simulink model "case1"  (R2024b)
settings: Solver=FixedStepAuto  StartTime=0  StopTime=1  FixedStep=1e-7  RelTol=1e-3
values from neighbouring files (symbols this model uses):
  SG_D_1_D = 0.01056    [IEEE9_case_parameters.m]    (also in case1_parameters.m; case2_parameters.m; case3_parameters.m; case4_parameters.m)
  SG_D_1_EnableSaturation = 0    [IEEE9_case_parameters.m]    (also in case1_parameters.m; case2_parameters.m; case3_parameters.m; case4_parameters.m)
  SG_D_1_f0 = 60    [IEEE9_case_parameters.m]    (also in case1_parameters.m; case2_parameters.m; case3_parameters.m; case4_parameters.m)
  SG_D_1_H = 7.5    [IEEE9_case_parameters.m]    (also in case1_parameters.m; case2_parameters.m; case3_parameters.m; case4_parameters.m)
  SG_D_1_K_A = 20    [IEEE9_case_parameters.m]    (also in case1_parameters.m; case2_parameters.m; case3_parameters.m; case4_parameters.m)
  SG_D_1_K_E = 1.000000e+1    (= 10)    [IEEE9_case_parameters.m]    (also in case1_parameters.m; case2_parameters.m; case3_parameters.m; case4_parameters.m)
  SG_D_1_K_F = 2.363    [IEEE9_case_parameters.m]    (also in case1_parameters.m; case2_parameters.m; case3_parameters.m; case4_parameters.m)
  SG_D_1_K_s = 0.5    [IEEE9_case_parameters.m]    (also in case1_parameters.m = 5; case2_parameters.m = 5; case3_parameters.m = 5; case4_parameters.m = 5)
  SG_D_1_R_a = 0.001088    [IEEE9_case_parameters.m]    (also in case1_parameters.m; case2_parameters.m; case3_parameters.m; case4_parameters.m)
  SG_D_1_S_A = 1    [IEEE9_case_parameters.m]    (also in case1_parameters.m; case2_parameters.m; case3_parameters.m; case4_parameters.m)
  SG_D_1_S_B = 0.103    [IEEE9_case_parameters.m]    (also in case1_parameters.m; case2_parameters.m; case3_parameters.m; case4_parameters.m)
  SG_D_1_S_N = 10.659857    [IEEE9_case_parameters.m]    (also in case1_parameters.m; case2_parameters.m; case3_parameters.m; case4_parameters.m)
  SG_D_1_SpeedPara = 200    [IEEE9_case_parameters.m]    (also in case1_parameters.m; case2_parameters.m; case3_parameters.m; case4_parameters.m)
  SG_D_1_T_0 = 0.720173    [IEEE9_case_parameters.m]    (also in case1_parameters.m = 0.755522; case2_parameters.m = 0.808931; case3_parameters.m = 0.869402; case4_parameters.m = 0.729316)
  SG_D_1_T_1 = 0.3    [IEEE9_case_parameters.m]    (also in case1_parameters.m; case2_parameters.m; case3_parameters.m; case4_parameters.m)
  SG_D_1_T_2 = 0.05    [IEEE9_case_parameters.m]    (also in case1_parameters.m; case2_parameters.m; case3_parameters.m; case4_parameters.m)
  SG_D_1_T_3 = 0.02    [IEEE9_case_parameters.m]    (also in case1_parameters.m; case2_parameters.m; case3_parameters.m; case4_parameters.m)
  SG_D_1_T_4 = 0.005    [IEEE9_case_parameters.m]    (also in case1_parameters.m; case2_parameters.m; case3_parameters.m; case4_parameters.m)
  SG_D_1_T_A = 0.02    [IEEE9_case_parameters.m]    (also in case1_parameters.m; case2_parameters.m; case3_parameters.m; case4_parameters.m)
  SG_D_1_T_dd = 8.000000e+0    (= 8)    [IEEE9_case_parameters.m]    (also in case1_parameters.m; case2_parameters.m; case3_parameters.m; case4_parameters.m)
  SG_D_1_T_ddd = 0.04    [IEEE9_case_parameters.m]    (also in case1_parameters.m; case2_parameters.m; case3_parameters.m; case4_parameters.m)
  SG_D_1_T_E = 0.314    [IEEE9_case_parameters.m]    (also in case1_parameters.m; case2_parameters.m; case3_parameters.m; case4_parameters.m)
  SG_D_1_T_F = 0.35    [IEEE9_case_parameters.m]    (also in case1_parameters.m; case2_parameters.m; case3_parameters.m; case4_parameters.m)
  SG_D_1_T_qd = 0.8    [IEEE9_case_parameters.m]    (also in case1_parameters.m; case2_parameters.m; case3_parameters.m; case4_parameters.m)
  SG_D_1_T_qdd = 0.02    [IEEE9_case_parameters.m]    (also in case1_parameters.m; case2_parameters.m; case3_parameters.m; case4_parameters.m)
  SG_D_1_T_speed = 0.1    [IEEE9_case_parameters.m]    (also in case1_parameters.m = 200; case2_parameters.m = 200; case3_parameters.m = 200; case4_parameters.m = 200)
  SG_D_1_T_w = 0.5    [IEEE9_case_parameters.m]    (also in case1_parameters.m; case2_parameters.m; case3_parameters.m; case4_parameters.m)
  SG_D_1_V_ref = 1.990276    [IEEE9_case_parameters.m]    (also in case1_parameters.m = 2.042296; case2_parameters.m = 2.051388; case3_parameters.m = 2.089584; case4_parameters.m = 2.01845)
  SG_D_1_w_ref = 376.991118    [IEEE9_case_parameters.m]    (also in case1_parameters.m; case2_parameters.m; case3_parameters.m; case4_parameters.m)
  SG_D_1_wb = 6.000000e+1    (= 60)    [IEEE9_case_parameters.m]    (also in case1_parameters.m; case2_parameters.m; case3_parameters.m; case4_parameters.m)
  SG_D_1_x_d = 1.9    [IEEE9_case_parameters.m]    (also in case1_parameters.m; case2_parameters.m; case3_parameters.m; case4_parameters.m)
  SG_D_1_x_dd = 0.302    [IEEE9_case_parameters.m]    (also in case1_parameters.m; case2_parameters.m; case3_parameters.m; case4_parameters.m)
  SG_D_1_x_ddd = 0.204    [IEEE9_case_parameters.m]    (also in case1_parameters.m; case2_parameters.m; case3_parameters.m; case4_parameters.m)
  SG_D_1_x_l = 0.05    [IEEE9_case_parameters.m]    (also in case1_parameters.m; case2_parameters.m; case3_parameters.m; case4_parameters.m)
  SG_D_1_x_q = 1.3    [IEEE9_case_parameters.m]    (also in case1_parameters.m; case2_parameters.m; case3_parameters.m; case4_parameters.m)
  SG_D_1_x_qd = 0.5    [IEEE9_case_parameters.m]    (also in case1_parameters.m; case2_parameters.m; case3_parameters.m; case4_parameters.m)
  SG_D_1_x_qdd = 0.3    [IEEE9_case_parameters.m]    (also in case1_parameters.m; case2_parameters.m; case3_parameters.m; case4_parameters.m)
  SG_D_2_D = 0.02    [IEEE9_case_parameters.m]    (also in case1_parameters.m; case2_parameters.m; case3_parameters.m; case4_parameters.m)
  SG_D_2_EnableSaturation = 0    [IEEE9_case_parameters.m]    (also in case1_parameters.m; case2_parameters.m; case3_parameters.m; case4_parameters.m)
  SG_D_2_f0 = 60    [IEEE9_case_parameters.m]    (also in case1_parameters.m; case2_parameters.m; case3_parameters.m; case4_parameters.m)
  SG_D_2_H = 8.000000e+0    (= 8)    [IEEE9_case_parameters.m]    (also in case1_parameters.m; case2_parameters.m; case3_parameters.m; case4_parameters.m)
  SG_D_2_K_A = 20    [IEEE9_case_parameters.m]    (also in case1_parameters.m; case2_parameters.m; case3_parameters.m; case4_parameters.m)
  SG_D_2_K_E = 1.000000e+1    (= 10)    [IEEE9_case_parameters.m]    (also in case1_parameters.m; case2_parameters.m; case3_parameters.m; case4_parameters.m)
  SG_D_2_K_F = 2.363    [IEEE9_case_parameters.m]    (also in case1_parameters.m; case2_parameters.m; case3_parameters.m; case4_parameters.m)
  SG_D_2_K_s = 0.5    [IEEE9_case_parameters.m]    (also in case1_parameters.m = 4; case2_parameters.m = 4; case3_parameters.m = 4; case4_parameters.m = 4)
  SG_D_2_R_a = 0.001088    [IEEE9_case_parameters.m]    (also in case1_parameters.m; case2_parameters.m; case3_parameters.m; case4_parameters.m)
  SG_D_2_S_A = 1    [IEEE9_case_parameters.m]    (also in case1_parameters.m; case2_parameters.m; case3_parameters.m; case4_parameters.m)
  SG_D_2_S_B = 0.103    [IEEE9_case_parameters.m]    (also in case1_parameters.m; case2_parameters.m; case3_parameters.m; case4_parameters.m)
  SG_D_2_S_N = 10.659857    [IEEE9_case_parameters.m]    (also in case1_parameters.m; case2_parameters.m; case3_parameters.m; case4_parameters.m)
  SG_D_2_SpeedPara = 200    [IEEE9_case_parameters.m]    (also in case1_parameters.m; case2_parameters.m; case3_parameters.m; case4_parameters.m)
  SG_D_2_T_0 = 1.632913    [IEEE9_case_parameters.m]    (also in case1_parameters.m = 1.632925; case2_parameters.m = 1.632915; case3_parameters.m = 1.632914; case4_parameters.m = 1.632927)
  SG_D_2_T_1 = 0.2    [IEEE9_case_parameters.m]    (also in case1_parameters.m; case2_parameters.m; case3_parameters.m; case4_parameters.m)
  SG_D_2_T_2 = 0.05    [IEEE9_case_parameters.m]    (also in case1_parameters.m; case2_parameters.m; case3_parameters.m; case4_parameters.m)
  SG_D_2_T_3 = 0.02    [IEEE9_case_parameters.m]    (also in case1_parameters.m; case2_parameters.m; case3_parameters.m; case4_parameters.m)
  SG_D_2_T_4 = 0.005    [IEEE9_case_parameters.m]    (also in case1_parameters.m; case2_parameters.m; case3_parameters.m; case4_parameters.m)
  SG_D_2_T_A = 0.02    [IEEE9_case_parameters.m]    (also in case1_parameters.m; case2_parameters.m; case3_parameters.m; case4_parameters.m)
  SG_D_2_T_dd = 7.9    [IEEE9_case_parameters.m]    (also in case1_parameters.m; case2_parameters.m; case3_parameters.m; case4_parameters.m)
  SG_D_2_T_ddd = 0.04    [IEEE9_case_parameters.m]    (also in case1_parameters.m; case2_parameters.m; case3_parameters.m; case4_parameters.m)
  SG_D_2_T_E = 0.314    [IEEE9_case_parameters.m]    (also in case1_parameters.m; case2_parameters.m; case3_parameters.m; case4_parameters.m)
  SG_D_2_T_F = 0.35    [IEEE9_case_parameters.m]    (also in case1_parameters.m; case2_parameters.m; case3_parameters.m; case4_parameters.m)
  SG_D_2_T_qd = 0.8    [IEEE9_case_parameters.m]    (also in case1_parameters.m; case2_parameters.m; case3_parameters.m; case4_parameters.m)
  SG_D_2_T_qdd = 0.015    [IEEE9_case_parameters.m]    (also in case1_parameters.m; case2_parameters.m; case3_parameters.m; case4_parameters.m)
  SG_D_2_T_speed = 0.1    [IEEE9_case_parameters.m]    (also in case1_parameters.m = 150; case2_parameters.m = 150; case3_parameters.m = 150; case4_parameters.m = 150)
  SG_D_2_T_w = 0.35    [IEEE9_case_parameters.m]    (also in case1_parameters.m; case2_parameters.m; case3_parameters.m; case4_parameters.m)
  SG_D_2_V_ref = 2.58547    [IEEE9_case_parameters.m]    (also in case1_parameters.m = 2.597896; case2_parameters.m = 2.587136; case3_parameters.m = 2.586042; case4_parameters.m = 2.599679)
  SG_D_2_w_ref = 376.991118    [IEEE9_case_parameters.m]    (also in case1_parameters.m; case2_parameters.m; case3_parameters.m; case4_parameters.m)
  SG_D_2_wb = 6.000000e+1    (= 60)    [IEEE9_case_parameters.m]    (also in case1_parameters.m; case2_parameters.m; case3_parameters.m; case4_parameters.m)
  SG_D_2_x_d = 1.8    [IEEE9_case_parameters.m]    (also in case1_parameters.m; case2_parameters.m; case3_parameters.m; case4_parameters.m)
  SG_D_2_x_dd = 0.302    [IEEE9_case_parameters.m]    (also in case1_parameters.m; case2_parameters.m; case3_parameters.m; case4_parameters.m)
  SG_D_2_x_ddd = 0.204    [IEEE9_case_parameters.m]    (also in case1_parameters.m; case2_parameters.m; case3_parameters.m; case4_parameters.m)
  SG_D_2_x_l = 0.05    [IEEE9_case_parameters.m]    (also in case1_parameters.m; case2_parameters.m; case3_parameters.m; case4_parameters.m)
  SG_D_2_x_q = 1.25    [IEEE9_case_parameters.m]    (also in case1_parameters.m; case2_parameters.m; case3_parameters.m; case4_parameters.m)
  SG_D_2_x_qd = 0.5    [IEEE9_case_parameters.m]    (also in case1_parameters.m; case2_parameters.m; case3_parameters.m; case4_parameters.m)
  SG_D_2_x_qdd = 0.3    [IEEE9_case_parameters.m]    (also in case1_parameters.m; case2_parameters.m; case3_parameters.m; case4_parameters.m)
  SG_D_3_D = 0.02    [IEEE9_case_parameters.m]    (also in case1_parameters.m; case2_parameters.m; case3_parameters.m; case4_parameters.m)
  SG_D_3_EnableSaturation = 0    [IEEE9_case_parameters.m]    (also in case1_parameters.m; case2_parameters.m; case3_parameters.m; case4_parameters.m)
  SG_D_3_f0 = 60    [IEEE9_case_parameters.m]    (also in case1_parameters.m; case2_parameters.m; case3_parameters.m; case4_parameters.m)
  SG_D_3_H = 7.7    [IEEE9_case_parameters.m]    (also in case1_parameters.m; case2_parameters.m; case3_parameters.m; case4_parameters.m)
  SG_D_3_K_A = 20    [IEEE9_case_parameters.m]    (also in case1_parameters.m; case2_parameters.m; case3_parameters.m; case4_parameters.m)
  SG_D_3_K_E = 1.000000e+1    (= 10)    [IEEE9_case_parameters.m]    (also in case1_parameters.m; case2_parameters.m; case3_parameters.m; case4_parameters.m)
  SG_D_3_K_F = 2.363    [IEEE9_case_parameters.m]    (also in case1_parameters.m; case2_parameters.m; case3_parameters.m; case4_parameters.m)
  SG_D_3_K_s = 0.2    [IEEE9_case_parameters.m]    (also in case1_parameters.m = 2; case2_parameters.m = 2; case3_parameters.m = 2; case4_parameters.m = 2)
  SG_D_3_R_a = 0.001088    [IEEE9_case_parameters.m]    (also in case1_parameters.m; case2_parameters.m; case3_parameters.m; case4_parameters.m)
  SG_D_3_S_A = 1    [IEEE9_case_parameters.m]    (also in case1_parameters.m; case2_parameters.m; case3_parameters.m; case4_parameters.m)
  SG_D_3_S_B = 0.103    [IEEE9_case_parameters.m]    (also in case1_parameters.m; case2_parameters.m; case3_parameters.m; case4_parameters.m)
  SG_D_3_S_N = 10.659857    [IEEE9_case_parameters.m]    (also in case1_parameters.m; case2_parameters.m; case3_parameters.m; case4_parameters.m)
  SG_D_3_SpeedPara = 200    [IEEE9_case_parameters.m]    (also in case1_parameters.m; case2_parameters.m; case3_parameters.m; case4_parameters.m)
  SG_D_3_T_0 = 0.850788    [IEEE9_case_parameters.m]    (also in case1_parameters.m = 0.850786; case2_parameters.m = 0.850787; case3_parameters.m; case4_parameters.m = 0.850786)
  SG_D_3_T_1 = 0.2    [IEEE9_case_parameters.m]    (also in case1_parameters.m; case2_parameters.m; case3_parameters.m; case4_parameters.m)
  SG_D_3_T_2 = 0.05    [IEEE9_case_parameters.m]    (also in case1_parameters.m; case2_parameters.m; case3_parameters.m; case4_parameters.m)
  SG_D_3_T_3 = 0.02    [IEEE9_case_parameters.m]    (also in case1_parameters.m; case2_parameters.m; case3_parameters.m; case4_parameters.m)
  SG_D_3_T_4 = 0.005    [IEEE9_case_parameters.m]    (also in case1_parameters.m; case2_parameters.m; case3_parameters.m; case4_parameters.m)
  SG_D_3_T_A = 0.02    [IEEE9_case_parameters.m]    (also in case1_parameters.m; case2_parameters.m; case3_parameters.m; case4_parameters.m)
  SG_D_3_T_dd = 8.1    [IEEE9_case_parameters.m]    (also in case1_parameters.m; case2_parameters.m; case3_parameters.m; case4_parameters.m)
  SG_D_3_T_ddd = 0.04    [IEEE9_case_parameters.m]    (also in case1_parameters.m; case2_parameters.m; case3_parameters.m; case4_parameters.m)
  SG_D_3_T_E = 0.314    [IEEE9_case_parameters.m]    (also in case1_parameters.m; case2_parameters.m; case3_parameters.m; case4_parameters.m)
  SG_D_3_T_F = 0.35    [IEEE9_case_parameters.m]    (also in case1_parameters.m; case2_parameters.m; case3_parameters.m; case4_parameters.m)
  SG_D_3_T_qd = 0.8    [IEEE9_case_parameters.m]    (also in case1_parameters.m; case2_parameters.m; case3_parameters.m; case4_parameters.m)
  SG_D_3_T_qdd = 0.015    [IEEE9_case_parameters.m]    (also in case1_parameters.m; case2_parameters.m; case3_parameters.m; case4_parameters.m)
  SG_D_3_T_speed = 0.1    [IEEE9_case_parameters.m]    (also in case1_parameters.m = 180; case2_parameters.m = 180; case3_parameters.m = 180; case4_parameters.m = 180)
  SG_D_3_T_w = 0.4    [IEEE9_case_parameters.m]    (also in case1_parameters.m; case2_parameters.m; case3_parameters.m; case4_parameters.m)
  SG_D_3_V_ref = 1.892727    [IEEE9_case_parameters.m]    (also in case1_parameters.m = 1.906439; case2_parameters.m = 1.895535; case3_parameters.m = 1.892105; case4_parameters.m = 1.906598)
  SG_D_3_w_ref = 376.991118    [IEEE9_case_parameters.m]    (also in case1_parameters.m; case2_parameters.m; case3_parameters.m; case4_parameters.m)
  SG_D_3_wb = 6.000000e+1    (= 60)    [IEEE9_case_parameters.m]    (also in case1_parameters.m; case2_parameters.m; case3_parameters.m; case4_parameters.m)
  SG_D_3_x_d = 1.85    [IEEE9_case_parameters.m]    (also in case1_parameters.m; case2_parameters.m; case3_parameters.m; case4_parameters.m)
  SG_D_3_x_dd = 0.302    [IEEE9_case_parameters.m]    (also in case1_parameters.m; case2_parameters.m; case3_parameters.m; case4_parameters.m)
  SG_D_3_x_ddd = 0.204    [IEEE9_case_parameters.m]    (also in case1_parameters.m; case2_parameters.m; case3_parameters.m; case4_parameters.m)
  SG_D_3_x_l = 0.05    [IEEE9_case_parameters.m]    (also in case1_parameters.m; case2_parameters.m; case3_parameters.m; case4_parameters.m)
  SG_D_3_x_q = 1.2    [IEEE9_case_parameters.m]    (also in case1_parameters.m; case2_parameters.m; case3_parameters.m; case4_parameters.m)
  SG_D_3_x_qd = 0.5    [IEEE9_case_parameters.m]    (also in case1_parameters.m; case2_parameters.m; case3_parameters.m; case4_parameters.m)
  SG_D_3_x_qdd = 0.3    [IEEE9_case_parameters.m]    (also in case1_parameters.m; case2_parameters.m; case3_parameters.m; case4_parameters.m)
(part 2 of 12)

== system case1/SG_D_2 ==
  v_d_SG_D_2 : Inport
  v_q_SG_D_2 : Inport  Port=2
  E_fd_SG_D_2 : Integrator  InitialCondition=3.195791296561274
  Px_1_SG_D_2 : Integrator  InitialCondition=0.0
  Px_2_SG_D_2 : Integrator  InitialCondition=0.0
  Px_3_SG_D_2 : Integrator  InitialCondition=7.086697555280228e-24
  R_f_SG_D_2 : Integrator  InitialCondition=21.576156667926544
  T_e_SG_D_2_block : Subsystem
  T_m_SG_D_2 : Integrator  InitialCondition=1.6329252190417882
  V_f_SG_D_2 : Integrator  InitialCondition=31.95791296561274
  d_E_fd_SG_D_2_block : Subsystem
  d_Px_1_SG_D_2_block : Subsystem
  d_Px_2_SG_D_2_block : Subsystem
  d_Px_3_SG_D_2_block : Subsystem
  d_R_f_SG_D_2_block : Subsystem
  d_T_m_SG_D_2_block : Subsystem
  d_V_f_SG_D_2_block : Subsystem
  d_psi_1d_SG_D_2_block : Subsystem
  d_psi_d_SG_D_2_block : Subsystem
  d_psi_fd_SG_D_2_block : Subsystem
  d_psi_gq_SG_D_2_block : Subsystem
  d_psi_kq_SG_D_2_block : Subsystem
  d_psi_q_SG_D_2_block : Subsystem
  d_theta_SG_D_2_block : Subsystem
  d_w_SG_D_2_block : Subsystem
  i_d_SG_D_2_block : Subsystem
  i_q_SG_D_2_block : Subsystem
  psi_1d_SG_D_2 : Integrator  InitialCondition=0.5903095464731192
  psi_d_SG_D_2 : Integrator  InitialCondition=0.5158672107563145
  psi_fd_SG_D_2 : Integrator  InitialCondition=0.9654989184858135
  psi_gq_SG_D_2 : Integrator  InitialCondition=0.5152428462796697
  psi_kq_SG_D_2 : Integrator  InitialCondition=-0.8243885540474714
  psi_q_SG_D_2 : Integrator  InitialCondition=-0.8587380771327827
  theta_SG_D_2 : Integrator  InitialCondition=1.1983532874479317
  theta_SG_D_2_out_block : Subsystem
  w_SG_D_2 : Integrator  InitialCondition=376.99111843077515
  w_SG_D_2_out_block : Subsystem
  i_d_SG_D_2 : Outport
  i_q_SG_D_2 : Outport  Port=2
  T_e_SG_D_2 : Outport  Port=3
  w_SG_D_2_out : Outport  Port=4
  theta_SG_D_2_out : Outport  Port=5
  wires:
  d_T_m_SG_D_2_block/1(Blockout_d_T_m_SG_D_2_43af5) -> T_m_SG_D_2/1
  T_e_SG_D_2_block/1(Blockout_T_e_SG_D_2_b65d9) -> T_e_SG_D_2/1
  d_Px_2_SG_D_2_block/1(Blockout_d_Px_2_SG_D_2_74daf) -> Px_2_SG_D_2/1
  w_SG_D_2/1 -> d_psi_d_SG_D_2_block/9(State_w_SG_D_2_46e5d), d_w_SG_D_2_block/1(State_w_SG_D_2_d69c3), d_V_f_SG_D_2_block/13(State_w_SG_D_2_2be4f), d_psi_q_SG_D_2_block/9(State_w_SG_D_2_df282), d_theta_SG_D_2_block/1(State_w_SG_D_2_5c0a1), d_Px_1_SG_D_2_block/2(State_w_SG_D_2_a2171), d_T_m_SG_D_2_block/1(State_w_SG_D_2_723fe), d_Px_3_SG_D_2_block/6(State_w_SG_D_2_a0c55), d_Px_2_SG_D_2_block/4(State_w_SG_D_2_d1507), d_V_f_SG_D_2_block/8(State_w_SG_D_2_bb1ed), w_SG_D_2_out_block/1(State_w_SG_D_2_39d84)
  d_Px_1_SG_D_2_block/1(Blockout_d_Px_1_SG_D_2_8641a) -> Px_1_SG_D_2/1
  d_theta_SG_D_2_block/1(Blockout_d_theta_SG_D_2_6c47c) -> theta_SG_D_2/1
  d_Px_3_SG_D_2_block/1(Blockout_d_Px_3_SG_D_2_3521b) -> Px_3_SG_D_2/1
  psi_q_SG_D_2/1 -> d_psi_d_SG_D_2_block/8(State_psi_q_SG_D_2_06491), d_psi_gq_SG_D_2_block/6(State_psi_q_SG_D_2_986ec), d_psi_gq_SG_D_2_block/9(State_psi_q_SG_D_2_b4e81), d_psi_kq_SG_D_2_block/5(State_psi_q_SG_D_2_af7b5), d_w_SG_D_2_block/6(State_psi_q_SG_D_2_041d5), d_V_f_SG_D_2_block/11(State_psi_q_SG_D_2_14f0d), d_psi_q_SG_D_2_block/3(State_psi_q_SG_D_2_34d65), i_d_SG_D_2_block/3(State_psi_q_SG_D_2_a8ffe), i_q_SG_D_2_block/3(State_psi_q_SG_D_2_008e1), T_e_SG_D_2_block/4(State_psi_q_SG_D_2_25b32), T_e_SG_D_2_block/5(State_psi_q_SG_D_2_fddea), d_V_f_SG_D_2_block/7(State_psi_q_SG_D_2_09452), d_w_SG_D_2_block/7(State_psi_q_SG_D_2_a083f)
  w_SG_D_2_out_block/1(Blockout_w_SG_D_2_out_2e2ba) -> w_SG_D_2_out/1
  psi_gq_SG_D_2/1 -> d_psi_q_SG_D_2_block/1(State_psi_gq_SG_D_2_52ba9), d_psi_gq_SG_D_2_block/2(State_psi_gq_SG_D_2_2d72f), d_psi_gq_SG_D_2_block/4(State_psi_gq_SG_D_2_96f10), d_V_f_SG_D_2_block/9(State_psi_gq_SG_D_2_56303), d_psi_gq_SG_D_2_block/1(State_psi_gq_SG_D_2_d4904), i_d_SG_D_2_block/1(State_psi_gq_SG_D_2_0a4ff), d_psi_kq_SG_D_2_block/3(State_psi_gq_SG_D_2_c1bff), d_psi_kq_SG_D_2_block/1(State_psi_gq_SG_D_2_b21d1), i_q_SG_D_2_block/1(State_psi_gq_SG_D_2_4b38b), d_w_SG_D_2_block/4(State_psi_gq_SG_D_2_37098), T_e_SG_D_2_block/2(State_psi_gq_SG_D_2_50ede), d_psi_gq_SG_D_2_block/7(State_psi_gq_SG_D_2_84d01)
  psi_fd_SG_D_2/1 -> d_psi_fd_SG_D_2_block/2(State_psi_fd_SG_D_2_87c43), d_psi_fd_SG_D_2_block/4(State_psi_fd_SG_D_2_c572b), d_psi_fd_SG_D_2_block/7(State_psi_fd_SG_D_2_150ec), d_psi_fd_SG_D_2_block/10(State_psi_fd_SG_D_2_9d902), d_psi_d_SG_D_2_block/3(State_psi_fd_SG_D_2_4d493), d_psi_1d_SG_D_2_block/5(State_psi_fd_SG_D_2_2bfe4), d_w_SG_D_2_block/10(State_psi_fd_SG_D_2_0ad40), d_psi_1d_SG_D_2_block/2(State_psi_fd_SG_D_2_d5601), i_d_SG_D_2_block/7(State_psi_fd_SG_D_2_62171), i_q_SG_D_2_block/7(State_psi_fd_SG_D_2_0701d), T_e_SG_D_2_block/8(State_psi_fd_SG_D_2_27f6e), d_V_f_SG_D_2_block/6(State_psi_fd_SG_D_2_7e9d1)
  Px_1_SG_D_2/1 -> d_Px_2_SG_D_2_block/2(State_Px_1_SG_D_2_4a486), d_Px_3_SG_D_2_block/4(State_Px_1_SG_D_2_19b2b), d_Px_3_SG_D_2_block/5(State_Px_1_SG_D_2_dcab9), d_Px_2_SG_D_2_block/3(State_Px_1_SG_D_2_0c9fb), d_Px_1_SG_D_2_block/1(State_Px_1_SG_D_2_dab25)
  psi_1d_SG_D_2/1 -> d_psi_fd_SG_D_2_block/3(State_psi_1d_SG_D_2_cf418), d_psi_fd_SG_D_2_block/5(State_psi_1d_SG_D_2_6822c), d_psi_fd_SG_D_2_block/8(State_psi_1d_SG_D_2_241cc), d_psi_d_SG_D_2_block/1(State_psi_1d_SG_D_2_48ea4), d_w_SG_D_2_block/8(State_psi_1d_SG_D_2_7d072), d_psi_1d_SG_D_2_block/3(State_psi_1d_SG_D_2_3af5a), d_psi_1d_SG_D_2_block/1(State_psi_1d_SG_D_2_96ec3), d_V_f_SG_D_2_block/4(State_psi_1d_SG_D_2_f4f15), i_d_SG_D_2_block/5(State_psi_1d_SG_D_2_a6845), i_q_SG_D_2_block/5(State_psi_1d_SG_D_2_4cf3f), T_e_SG_D_2_block/6(State_psi_1d_SG_D_2_6821c)
  i_d_SG_D_2_block/1(Blockout_i_d_SG_D_2_76c8b) -> i_d_SG_D_2/1
  psi_d_SG_D_2/1 -> d_psi_d_SG_D_2_block/2(State_psi_d_SG_D_2_8d25d), d_psi_1d_SG_D_2_block/4(State_psi_d_SG_D_2_4d81a), i_d_SG_D_2_block/6(State_psi_d_SG_D_2_bb259), d_psi_q_SG_D_2_block/8(State_psi_d_SG_D_2_1d0f8), d_V_f_SG_D_2_block/12(State_psi_d_SG_D_2_84408), d_psi_fd_SG_D_2_block/9(State_psi_d_SG_D_2_887e8), d_w_SG_D_2_block/9(State_psi_d_SG_D_2_8384e), d_w_SG_D_2_block/3(State_psi_d_SG_D_2_3a37a), i_q_SG_D_2_block/6(State_psi_d_SG_D_2_91eea), d_V_f_SG_D_2_block/5(State_psi_d_SG_D_2_39d83), d_psi_fd_SG_D_2_block/6(State_psi_d_SG_D_2_85721), T_e_SG_D_2_block/1(State_psi_d_SG_D_2_d17d7), T_e_SG_D_2_block/7(State_psi_d_SG_D_2_3bce2)
  psi_kq_SG_D_2/1 -> d_psi_q_SG_D_2_block/2(State_psi_kq_SG_D_2_a91e4), d_psi_gq_SG_D_2_block/3(State_psi_kq_SG_D_2_8efed), d_psi_gq_SG_D_2_block/5(State_psi_kq_SG_D_2_f03b3), d_psi_kq_SG_D_2_block/2(State_psi_kq_SG_D_2_91d69), d_psi_gq_SG_D_2_block/8(State_psi_kq_SG_D_2_c2c6b), d_psi_kq_SG_D_2_block/4(State_psi_kq_SG_D_2_611bb), i_d_SG_D_2_block/2(State_psi_kq_SG_D_2_7acfc), i_q_SG_D_2_block/2(State_psi_kq_SG_D_2_d6d60), d_V_f_SG_D_2_block/10(State_psi_kq_SG_D_2_82247), d_w_SG_D_2_block/5(State_psi_kq_SG_D_2_af83b), T_e_SG_D_2_block/3(State_psi_kq_SG_D_2_ad282)
  v_d_SG_D_2/1 -> d_psi_d_SG_D_2_block/4(Input_v_d_SG_D_2_e74d4), d_psi_q_SG_D_2_block/4(Input_v_d_SG_D_2_5ea16)
  T_m_SG_D_2/1 -> d_T_m_SG_D_2_block/2(State_T_m_SG_D_2_d95aa), d_w_SG_D_2_block/2(State_T_m_SG_D_2_7a8a9)
  d_V_f_SG_D_2_block/1(Blockout_d_V_f_SG_D_2_347d2) -> V_f_SG_D_2/1
  v_q_SG_D_2/1 -> d_psi_d_SG_D_2_block/6(Input_v_q_SG_D_2_ef7b1), d_psi_q_SG_D_2_block/6(Input_v_q_SG_D_2_1b817)
  Px_2_SG_D_2/1 -> d_Px_2_SG_D_2_block/1(State_Px_2_SG_D_2_5b382), d_Px_3_SG_D_2_block/3(State_Px_2_SG_D_2_7bb9c), d_Px_3_SG_D_2_block/2(State_Px_2_SG_D_2_29f59)
  theta_SG_D_2/1 -> d_psi_q_SG_D_2_block/5(State_theta_SG_D_2_2fc52), i_d_SG_D_2_block/8(State_theta_SG_D_2_f5053), i_q_SG_D_2_block/8(State_theta_SG_D_2_18733), i_q_SG_D_2_block/4(State_theta_SG_D_2_18eff), theta_SG_D_2_out_block/1(State_theta_SG_D_2_2515d), i_d_SG_D_2_block/4(State_theta_SG_D_2_c8d9f), d_psi_d_SG_D_2_block/7(State_theta_SG_D_2_069cc), d_psi_q_SG_D_2_block/7(State_theta_SG_D_2_f1308), d_psi_d_SG_D_2_block/5(State_theta_SG_D_2_cb884)
  d_psi_1d_SG_D_2_block/1(Blockout_d_psi_1d_SG_D_2_57022) -> psi_1d_SG_D_2/1
  d_R_f_SG_D_2_block/1(Blockout_d_R_f_SG_D_2_3f1f3) -> R_f_SG_D_2/1
  R_f_SG_D_2/1 -> d_V_f_SG_D_2_block/2(State_R_f_SG_D_2_e5370), d_R_f_SG_D_2_block/2(State_R_f_SG_D_2_6bf16)
  theta_SG_D_2_out_block/1(Blockout_theta_SG_D_2_out_503d1) -> theta_SG_D_2_out/1
  d_psi_gq_SG_D_2_block/1(Blockout_d_psi_gq_SG_D_2_f38dc) -> psi_gq_SG_D_2/1
  d_psi_d_SG_D_2_block/1(Blockout_d_psi_d_SG_D_2_591f5) -> psi_d_SG_D_2/1
  d_w_SG_D_2_block/1(Blockout_d_w_SG_D_2_dff9f) -> w_SG_D_2/1
  d_psi_q_SG_D_2_block/1(Blockout_d_psi_q_SG_D_2_5eec6) -> psi_q_SG_D_2/1
  d_psi_kq_SG_D_2_block/1(Blockout_d_psi_kq_SG_D_2_4ff78) -> psi_kq_SG_D_2/1
  i_q_SG_D_2_block/1(Blockout_i_q_SG_D_2_02eb4) -> i_q_SG_D_2/1
  V_f_SG_D_2/1 -> d_V_f_SG_D_2_block/14(State_V_f_SG_D_2_eb789), d_E_fd_SG_D_2_block/2(State_V_f_SG_D_2_853e9)
  Px_3_SG_D_2/1 -> d_V_f_SG_D_2_block/3(State_Px_3_SG_D_2_3a9e9), d_Px_3_SG_D_2_block/1(State_Px_3_SG_D_2_47d77)
  d_E_fd_SG_D_2_block/1(Blockout_d_E_fd_SG_D_2_6e556) -> E_fd_SG_D_2/1
  E_fd_SG_D_2/1 -> d_V_f_SG_D_2_block/1(State_E_fd_SG_D_2_4dd56), d_R_f_SG_D_2_block/1(State_E_fd_SG_D_2_b3245), d_psi_fd_SG_D_2_block/1(State_E_fd_SG_D_2_9c9d0), d_E_fd_SG_D_2_block/1(State_E_fd_SG_D_2_f3b44)
  d_psi_fd_SG_D_2_block/1(Blockout_d_psi_fd_SG_D_2_b0c7a) -> psi_fd_SG_D_2/1

== system case1/SG_D_3 ==
  v_d_SG_D_3 : Inport
  v_q_SG_D_3 : Inport  Port=2
  E_fd_SG_D_3 : Integrator  InitialCondition=1.8128770595240795
  Px_1_SG_D_3 : Integrator  InitialCondition=0.0
  Px_2_SG_D_3 : Integrator  InitialCondition=0.0
  Px_3_SG_D_3 : Integrator  InitialCondition=5.5764488625501145e-24
  R_f_SG_D_3 : Integrator  InitialCondition=12.239509976158287
  T_e_SG_D_3_block : Subsystem
  T_m_SG_D_3 : Integrator  InitialCondition=0.8507861887621803
  V_f_SG_D_3 : Integrator  InitialCondition=18.1287705952408
  d_E_fd_SG_D_3_block : Subsystem
  d_Px_1_SG_D_3_block : Subsystem
  d_Px_2_SG_D_3_block : Subsystem
  d_Px_3_SG_D_3_block : Subsystem
  d_R_f_SG_D_3_block : Subsystem
  d_T_m_SG_D_3_block : Subsystem
  d_V_f_SG_D_3_block : Subsystem
  d_psi_1d_SG_D_3_block : Subsystem
  d_psi_d_SG_D_3_block : Subsystem
  d_psi_fd_SG_D_3_block : Subsystem
  d_psi_gq_SG_D_3_block : Subsystem
  d_psi_kq_SG_D_3_block : Subsystem
  d_psi_q_SG_D_3_block : Subsystem
  d_theta_SG_D_3_block : Subsystem
  d_w_SG_D_3_block : Subsystem
  i_d_SG_D_3_block : Subsystem
  i_q_SG_D_3_block : Subsystem
  psi_1d_SG_D_3 : Integrator  InitialCondition=0.7269094989362452
  psi_d_SG_D_3 : Integrator  InitialCondition=0.6967437333643608
  psi_fd_SG_D_3 : Integrator  InitialCondition=0.8789449574185421
  psi_gq_SG_D_3 : Integrator  InitialCondition=0.419188473974919
  psi_kq_SG_D_3 : Integrator  InitialCondition=-0.6886667786730812
  psi_q_SG_D_3 : Integrator  InitialCondition=-0.7186088125284327
  theta_SG_D_3 : Integrator  InitialCondition=0.88169001906526
  theta_SG_D_3_out_block : Subsystem
  w_SG_D_3 : Integrator  InitialCondition=376.99111843077515
  w_SG_D_3_out_block : Subsystem
  i_d_SG_D_3 : Outport
  i_q_SG_D_3 : Outport  Port=2
  T_e_SG_D_3 : Outport  Port=3
  w_SG_D_3_out : Outport  Port=4
  theta_SG_D_3_out : Outport  Port=5
  wires:
  d_Px_1_SG_D_3_block/1(Blockout_d_Px_1_SG_D_3_617e0) -> Px_1_SG_D_3/1
  w_SG_D_3/1 -> d_V_f_SG_D_3_block/13(State_w_SG_D_3_e4083), d_w_SG_D_3_block/1(State_w_SG_D_3_f2997), d_V_f_SG_D_3_block/8(State_w_SG_D_3_c73a4), d_psi_d_SG_D_3_block/9(State_w_SG_D_3_2ec24), d_theta_SG_D_3_block/1(State_w_SG_D_3_f4ecf), d_Px_1_SG_D_3_block/2(State_w_SG_D_3_e1b7a), d_Px_2_SG_D_3_block/4(State_w_SG_D_3_b1950), d_Px_3_SG_D_3_block/6(State_w_SG_D_3_60df7), d_T_m_SG_D_3_block/1(State_w_SG_D_3_66142), w_SG_D_3_out_block/1(State_w_SG_D_3_cb7ae), d_psi_q_SG_D_3_block/9(State_w_SG_D_3_33157)
  d_T_m_SG_D_3_block/1(Blockout_d_T_m_SG_D_3_67a05) -> T_m_SG_D_3/1
  R_f_SG_D_3/1 -> d_V_f_SG_D_3_block/2(State_R_f_SG_D_3_73220), d_R_f_SG_D_3_block/2(State_R_f_SG_D_3_7f0e0)
  w_SG_D_3_out_block/1(Blockout_w_SG_D_3_out_7c137) -> w_SG_D_3_out/1
  d_Px_2_SG_D_3_block/1(Blockout_d_Px_2_SG_D_3_63947) -> Px_2_SG_D_3/1
  d_w_SG_D_3_block/1(Blockout_d_w_SG_D_3_f936a) -> w_SG_D_3/1
  Px_1_SG_D_3/1 -> d_Px_1_SG_D_3_block/1(State_Px_1_SG_D_3_d0b1d), d_Px_2_SG_D_3_block/3(State_Px_1_SG_D_3_ad022), d_Px_3_SG_D_3_block/5(State_Px_1_SG_D_3_ac5bc), d_Px_3_SG_D_3_block/4(State_Px_1_SG_D_3_57193), d_Px_2_SG_D_3_block/2(State_Px_1_SG_D_3_f2f90)
  d_theta_SG_D_3_block/1(Blockout_d_theta_SG_D_3_d61c2) -> theta_SG_D_3/1
  d_Px_3_SG_D_3_block/1(Blockout_d_Px_3_SG_D_3_2448a) -> Px_3_SG_D_3/1
  T_m_SG_D_3/1 -> d_T_m_SG_D_3_block/2(State_T_m_SG_D_3_24b45), d_w_SG_D_3_block/2(State_T_m_SG_D_3_65f4a)
  psi_q_SG_D_3/1 -> d_psi_q_SG_D_3_block/3(State_psi_q_SG_D_3_1c339), d_w_SG_D_3_block/7(State_psi_q_SG_D_3_24df4), d_V_f_SG_D_3_block/7(State_psi_q_SG_D_3_f59ba), d_w_SG_D_3_block/6(State_psi_q_SG_D_3_7f5a7), d_psi_kq_SG_D_3_block/5(State_psi_q_SG_D_3_3b888), d_psi_d_SG_D_3_block/8(State_psi_q_SG_D_3_aaa02), d_V_f_SG_D_3_block/11(State_psi_q_SG_D_3_dedb4), i_d_SG_D_3_block/3(State_psi_q_SG_D_3_bb946), T_e_SG_D_3_block/4(State_psi_q_SG_D_3_ebc14), T_e_SG_D_3_block/5(State_psi_q_SG_D_3_fe94c), d_psi_gq_SG_D_3_block/6(State_psi_q_SG_D_3_b8378), i_q_SG_D_3_block/3(State_psi_q_SG_D_3_dc7e8), d_psi_gq_SG_D_3_block/9(State_psi_q_SG_D_3_1463f)
  psi_gq_SG_D_3/1 -> d_psi_q_SG_D_3_block/1(State_psi_gq_SG_D_3_b4a4d), d_psi_gq_SG_D_3_block/1(State_psi_gq_SG_D_3_67c62), d_psi_gq_SG_D_3_block/2(State_psi_gq_SG_D_3_5cce3), d_psi_gq_SG_D_3_block/7(State_psi_gq_SG_D_3_e3684), d_V_f_SG_D_3_block/9(State_psi_gq_SG_D_3_a694f), d_w_SG_D_3_block/4(State_psi_gq_SG_D_3_d1af9), i_d_SG_D_3_block/1(State_psi_gq_SG_D_3_aa812), d_psi_kq_SG_D_3_block/1(State_psi_gq_SG_D_3_d2333), i_q_SG_D_3_block/1(State_psi_gq_SG_D_3_49972), d_psi_gq_SG_D_3_block/4(State_psi_gq_SG_D_3_55580), d_psi_kq_SG_D_3_block/3(State_psi_gq_SG_D_3_852d7), T_e_SG_D_3_block/2(State_psi_gq_SG_D_3_86cef)
  theta_SG_D_3/1 -> d_psi_d_SG_D_3_block/5(State_theta_SG_D_3_ff733), d_psi_q_SG_D_3_block/5(State_theta_SG_D_3_b412e), i_d_SG_D_3_block/8(State_theta_SG_D_3_03ed0), d_psi_q_SG_D_3_block/7(State_theta_SG_D_3_6cd7f), i_q_SG_D_3_block/8(State_theta_SG_D_3_713df), theta_SG_D_3_out_block/1(State_theta_SG_D_3_1872a), i_q_SG_D_3_block/4(State_theta_SG_D_3_30883), d_psi_d_SG_D_3_block/7(State_theta_SG_D_3_0d41b), i_d_SG_D_3_block/4(State_theta_SG_D_3_b0af7)
  psi_d_SG_D_3/1 -> d_psi_fd_SG_D_3_block/9(State_psi_d_SG_D_3_9355f), d_psi_q_SG_D_3_block/8(State_psi_d_SG_D_3_39242), d_psi_1d_SG_D_3_block/4(State_psi_d_SG_D_3_fc886), d_w_SG_D_3_block/9(State_psi_d_SG_D_3_99f2e), i_q_SG_D_3_block/6(State_psi_d_SG_D_3_ab8d9), d_V_f_SG_D_3_block/5(State_psi_d_SG_D_3_e0bb1), T_e_SG_D_3_block/1(State_psi_d_SG_D_3_e2290), i_d_SG_D_3_block/6(State_psi_d_SG_D_3_8ce12), T_e_SG_D_3_block/7(State_psi_d_SG_D_3_4b90d), d_V_f_SG_D_3_block/12(State_psi_d_SG_D_3_f76a9), d_psi_fd_SG_D_3_block/6(State_psi_d_SG_D_3_67b18), d_w_SG_D_3_block/3(State_psi_d_SG_D_3_22dab), d_psi_d_SG_D_3_block/2(State_psi_d_SG_D_3_98be9)
  v_d_SG_D_3/1 -> d_psi_q_SG_D_3_block/4(Input_v_d_SG_D_3_3c95f), d_psi_d_SG_D_3_block/4(Input_v_d_SG_D_3_1db53)
  v_q_SG_D_3/1 -> d_psi_d_SG_D_3_block/6(Input_v_q_SG_D_3_da623), d_psi_q_SG_D_3_block/6(Input_v_q_SG_D_3_30458)
  Px_2_SG_D_3/1 -> d_Px_2_SG_D_3_block/1(State_Px_2_SG_D_3_42098), d_Px_3_SG_D_3_block/2(State_Px_2_SG_D_3_9be0b), d_Px_3_SG_D_3_block/3(State_Px_2_SG_D_3_dd0dd)
  psi_kq_SG_D_3/1 -> d_psi_q_SG_D_3_block/2(State_psi_kq_SG_D_3_e7fae), d_psi_gq_SG_D_3_block/3(State_psi_kq_SG_D_3_3a689), d_psi_gq_SG_D_3_block/5(State_psi_kq_SG_D_3_bd2f5), d_psi_gq_SG_D_3_block/8(State_psi_kq_SG_D_3_98fbc), d_psi_kq_SG_D_3_block/2(State_psi_kq_SG_D_3_6b251), d_w_SG_D_3_block/5(State_psi_kq_SG_D_3_1f4e8), d_V_f_SG_D_3_block/10(State_psi_kq_SG_D_3_b1cec), d_psi_kq_SG_D_3_block/4(State_psi_kq_SG_D_3_8c307), i_q_SG_D_3_block/2(State_psi_kq_SG_D_3_db825), i_d_SG_D_3_block/2(State_psi_kq_SG_D_3_86816), T_e_SG_D_3_block/3(State_psi_kq_SG_D_3_cb0a5)
  psi_fd_SG_D_3/1 -> d_psi_fd_SG_D_3_block/2(State_psi_fd_SG_D_3_c9fb1), d_psi_fd_SG_D_3_block/7(State_psi_fd_SG_D_3_ae38b), d_psi_fd_SG_D_3_block/10(State_psi_fd_SG_D_3_ccc41), d_psi_fd_SG_D_3_block/4(State_psi_fd_SG_D_3_fd18f), d_psi_d_SG_D_3_block/3(State_psi_fd_SG_D_3_efb9b), d_psi_1d_SG_D_3_block/2(State_psi_fd_SG_D_3_10bdc), d_psi_1d_SG_D_3_block/5(State_psi_fd_SG_D_3_12757), d_w_SG_D_3_block/10(State_psi_fd_SG_D_3_82d9b), d_V_f_SG_D_3_block/6(State_psi_fd_SG_D_3_3fc20), i_d_SG_D_3_block/7(State_psi_fd_SG_D_3_34c08), i_q_SG_D_3_block/7(State_psi_fd_SG_D_3_ce3ba), T_e_SG_D_3_block/8(State_psi_fd_SG_D_3_9749b)
  d_psi_kq_SG_D_3_block/1(Blockout_d_psi_kq_SG_D_3_28baf) -> psi_kq_SG_D_3/1
  psi_1d_SG_D_3/1 -> d_psi_fd_SG_D_3_block/3(State_psi_1d_SG_D_3_61581), d_psi_fd_SG_D_3_block/5(State_psi_1d_SG_D_3_9f27e), d_psi_fd_SG_D_3_block/8(State_psi_1d_SG_D_3_5274a), d_psi_d_SG_D_3_block/1(State_psi_1d_SG_D_3_a5cf0), d_psi_1d_SG_D_3_block/1(State_psi_1d_SG_D_3_697cb), d_psi_1d_SG_D_3_block/3(State_psi_1d_SG_D_3_13000), d_w_SG_D_3_block/8(State_psi_1d_SG_D_3_fafae), d_V_f_SG_D_3_block/4(State_psi_1d_SG_D_3_daa8b), i_d_SG_D_3_block/5(State_psi_1d_SG_D_3_8f98b), i_q_SG_D_3_block/5(State_psi_1d_SG_D_3_0bea5), T_e_SG_D_3_block/6(State_psi_1d_SG_D_3_b91a5)
  theta_SG_D_3_out_block/1(Blockout_theta_SG_D_3_out_50464) -> theta_SG_D_3_out/1
  d_V_f_SG_D_3_block/1(Blockout_d_V_f_SG_D_3_85a9a) -> V_f_SG_D_3/1
  d_psi_d_SG_D_3_block/1(Blockout_d_psi_d_SG_D_3_cc8c1) -> psi_d_SG_D_3/1
  i_d_SG_D_3_block/1(Blockout_i_d_SG_D_3_90043) -> i_d_SG_D_3/1
  i_q_SG_D_3_block/1(Blockout_i_q_SG_D_3_22201) -> i_q_SG_D_3/1
  d_psi_q_SG_D_3_block/1(Blockout_d_psi_q_SG_D_3_3a763) -> psi_q_SG_D_3/1
  d_R_f_SG_D_3_block/1(Blockout_d_R_f_SG_D_3_113ff) -> R_f_SG_D_3/1
  d_psi_1d_SG_D_3_block/1(Blockout_d_psi_1d_SG_D_3_1ecde) -> psi_1d_SG_D_3/1
  d_psi_gq_SG_D_3_block/1(Blockout_d_psi_gq_SG_D_3_ef58c) -> psi_gq_SG_D_3/1
  T_e_SG_D_3_block/1(Blockout_T_e_SG_D_3_5971a) -> T_e_SG_D_3/1
  V_f_SG_D_3/1 -> d_E_fd_SG_D_3_block/2(State_V_f_SG_D_3_378e4), d_V_f_SG_D_3_block/14(State_V_f_SG_D_3_b01ff)
  Px_3_SG_D_3/1 -> d_V_f_SG_D_3_block/3(State_Px_3_SG_D_3_ece11), d_Px_3_SG_D_3_block/1(State_Px_3_SG_D_3_e3475)
  d_E_fd_SG_D_3_block/1(Blockout_d_E_fd_SG_D_3_6f2ed) -> E_fd_SG_D_3/1
  E_fd_SG_D_3/1 -> d_R_f_SG_D_3_block/1(State_E_fd_SG_D_3_666b5), d_psi_fd_SG_D_3_block/1(State_E_fd_SG_D_3_02b0a), d_V_f_SG_D_3_block/1(State_E_fd_SG_D_3_3245d), d_E_fd_SG_D_3_block/1(State_E_fd_SG_D_3_b50ae)
  d_psi_fd_SG_D_3_block/1(Blockout_d_psi_fd_SG_D_3_01811) -> psi_fd_SG_D_3/1

== system case1/AC_1/d_id_line_1_4_block ==
  note: d_id_line_1_4 in case1
      | $376.991118430775\,\mathrm{iq}_{\mathrm{line},1,4}+6387.9543042679\,\mathrm{vd}_{\mathrm{bus},1}-6387.9543042679\,\mathrm{vd}_{\mathrm{bus},4}$
      | Automatically generated on 2025-10-31 18:50:42 .
  State_iq_line_1_4_1aaa5 : Inport
  State_vd_bus_1_63720 : Inport  Port=2
  State_vd_bus_4_e2161 : Inport  Port=3
  Add_60d5f : Sum
  Constant_376.991118430775_1db3d : Constant  Value=376.991118430775
  Constant_6387.9543042679_5cc9b : Constant  Value=6387.9543042679
  Constant_6387.9543042679_779ca : Constant  Value=6387.9543042679
  Product_135a9 : Product
  Product_5f307 : Product
  Product_cfe0e : Product
  Subtract_40cfb : Sum  Inputs=+-
  Blockout_d_id_line_1_4_02e23 : Outport
  wires:
  Constant_376.991118430775_1db3d/1 -> Product_135a9/1
  Product_5f307/1 -> Add_60d5f/2
  State_iq_line_1_4_1aaa5/1 -> Product_135a9/2
  Subtract_40cfb/1 -> Blockout_d_id_line_1_4_02e23/1
  Constant_6387.9543042679_779ca/1 -> Product_5f307/1
  Product_135a9/1 -> Add_60d5f/1
  State_vd_bus_1_63720/1 -> Product_5f307/2
  Constant_6387.9543042679_5cc9b/1 -> Product_cfe0e/1
  State_vd_bus_4_e2161/1 -> Product_cfe0e/2
  Add_60d5f/1 -> Subtract_40cfb/1
  Product_cfe0e/1 -> Subtract_40cfb/2

== system case1/AC_1/d_id_line_3_6_block ==
  note: d_id_line_3_6 in case1
      | $376.991118430775\,\mathrm{iq}_{\mathrm{line},3,6}+6278.9448451507\,\mathrm{vd}_{\mathrm{bus},3}-6278.9448451507\,\mathrm{vd}_{\mathrm{bus},6}$
      | Automatically generated on 2025-10-31 18:50:49 .
  State_iq_line_3_6_218be : Inport
  State_vd_bus_3_5f170 : Inport  Port=2
  State_vd_bus_6_af45e : Inport  Port=3
  Add_84dba : Sum
  Constant_376.991118430775_d7f55 : Constant  Value=376.991118430775
  Constant_6278.9448451507_1ef3b : Constant  Value=6278.9448451507
  Constant_6278.9448451507_255f9 : Constant  Value=6278.9448451507
  Product_0e620 : Product
  Product_e4657 : Product
  Product_f425f : Product
  Subtract_358f5 : Sum  Inputs=+-
  Blockout_d_id_line_3_6_44702 : Outport
  wires:
  State_vd_bus_3_5f170/1 -> Product_e4657/2
  Constant_376.991118430775_d7f55/1 -> Product_0e620/1
  Product_e4657/1 -> Add_84dba/2
  State_iq_line_3_6_218be/1 -> Product_0e620/2
  Constant_6278.9448451507_255f9/1 -> Product_e4657/1
  Product_0e620/1 -> Add_84dba/1
  Constant_6278.9448451507_1ef3b/1 -> Product_f425f/1
  State_vd_bus_6_af45e/1 -> Product_f425f/2
  Add_84dba/1 -> Subtract_358f5/1
  Product_f425f/1 -> Subtract_358f5/2
  Subtract_358f5/1 -> Blockout_d_id_line_3_6_44702/1

== system case1/AC_1/d_id_line_4_5_block ==
  note: d_id_line_4_5 in case1
      | $376.991118430775\,\mathrm{iq}_{\mathrm{line},4,5}-70.7030565753656\,\mathrm{id}_{\mathrm{line},4,5}+3999.41486875903\,\mathrm{vd}_{\mathrm{bus},4}-3999.41486875903\,\mathrm{vd}_{\mathrm{bus},5}$
      | Automatically generated on 2025-10-31 18:50:44 .
  State_id_line_4_5_2f9d9 : Inport
  State_iq_line_4_5_28448 : Inport  Port=2
  State_vd_bus_4_1e1bc : Inport  Port=3
  State_vd_bus_5_d1c47 : Inport  Port=4
  Add_6c9bc : Sum
  Add_a2d7a : Sum
  Constant_-70.7030565753656_ecf79 : Constant  Value=-70.7030565753656
  Constant_376.991118430775_057fa : Constant  Value=376.991118430775
  Constant_3999.41486875903_331d7 : Constant  Value=3999.41486875903
  Constant_3999.41486875903_4c308 : Constant  Value=3999.41486875903
  Product_20dd3 : Product
  Product_40b8d : Product
  Product_4ab11 : Product
  Product_851e1 : Product
  Subtract_d7ca6 : Sum  Inputs=+-
  Blockout_d_id_line_4_5_a9a06 : Outport
  wires:
  Constant_-70.7030565753656_ecf79/1 -> Product_20dd3/1
  Product_4ab11/1 -> Add_a2d7a/2
  State_id_line_4_5_2f9d9/1 -> Product_20dd3/2
  Constant_376.991118430775_057fa/1 -> Product_4ab11/1
  State_iq_line_4_5_28448/1 -> Product_4ab11/2
  Product_20dd3/1 -> Add_a2d7a/1
  Constant_3999.41486875903_331d7/1 -> Product_40b8d/1
  State_vd_bus_4_1e1bc/1 -> Product_40b8d/2
  Add_a2d7a/1 -> Add_6c9bc/1
  Product_40b8d/1 -> Add_6c9bc/2
  Constant_3999.41486875903_4c308/1 -> Product_851e1/1
  State_vd_bus_5_d1c47/1 -> Product_851e1/2
  Add_6c9bc/1 -> Subtract_d7ca6/1
  Product_851e1/1 -> Subtract_d7ca6/2
  Subtract_d7ca6/1 -> Blockout_d_id_line_4_5_a9a06/1

== system case1/AC_1/d_id_line_5_6_block ==
  note: d_id_line_5_6 in case1
      | $376.991118430775\,\mathrm{iq}_{\mathrm{line},5,6}-87.7794349454712\,\mathrm{id}_{\mathrm{line},5,6}+2164.38922309312\,\mathrm{vd}_{\mathrm{bus},5}-2164.38922309312\,\mathrm{vd}_{\mathrm{bus},6}$
      | Automatically generated on 2025-10-31 18:50:47 .
  State_id_line_5_6_678c2 : Inport
  State_iq_line_5_6_30e91 : Inport  Port=2
  State_vd_bus_5_4803e : Inport  Port=3
  State_vd_bus_6_fd499 : Inport  Port=4
  Add_dc02f : Sum
  Add_f4c2c : Sum
  Constant_-87.7794349454712_5ecac : Constant  Value=-87.7794349454712
  Constant_2164.38922309312_b183c : Constant  Value=2164.38922309312
  Constant_2164.38922309312_fd1af : Constant  Value=2164.38922309312
  Constant_376.991118430775_8f566 : Constant  Value=376.991118430775
  Product_01e49 : Product
  Product_0aa63 : Product
  Product_3d5de : Product
  Product_5b84d : Product
  Subtract_14836 : Sum  Inputs=+-
  Blockout_d_id_line_5_6_1f7ce : Outport
  wires:
  Constant_-87.7794349454712_5ecac/1 -> Product_0aa63/1
  Product_01e49/1 -> Add_f4c2c/2
  State_id_line_5_6_678c2/1 -> Product_0aa63/2
  Constant_376.991118430775_8f566/1 -> Product_01e49/1
  Product_0aa63/1 -> Add_f4c2c/1
  State_iq_line_5_6_30e91/1 -> Product_01e49/2
  Constant_2164.38922309312_b183c/1 -> Product_3d5de/1
  Product_5b84d/1 -> Subtract_14836/2
  State_vd_bus_5_4803e/1 -> Product_3d5de/2
  Add_f4c2c/1 -> Add_dc02f/1
  Product_3d5de/1 -> Add_dc02f/2
  Constant_2164.38922309312_fd1af/1 -> Product_5b84d/1
  State_vd_bus_6_fd499/1 -> Product_5b84d/2
  Add_dc02f/1 -> Subtract_14836/1
  Subtract_14836/1 -> Blockout_d_id_line_5_6_1f7ce/1

== system case1/AC_1/d_id_line_6_7_block ==
  note: d_id_line_6_7 in case1
      | $376.991118430775\,\mathrm{iq}_{\mathrm{line},6,7}-45.1713972564836\,\mathrm{id}_{\mathrm{line},6,7}+3650.2596024388\,\mathrm{vd}_{\mathrm{bus},6}-3650.2596024388\,\mathrm{vd}_{\mathrm{bus},7}$
      | Automatically generated on 2025-10-31 18:50:51 .
  State_id_line_6_7_fdc4e : Inport
  State_iq_line_6_7_9688a : Inport  Port=2
  State_vd_bus_6_febc2 : Inport  Port=3
  State_vd_bus_7_50435 : Inport  Port=4
  Add_112c4 : Sum
  Add_f2513 : Sum
  Constant_-45.1713972564836_0ad27 : Constant  Value=-45.1713972564836
  Constant_3650.2596024388_c2f5c : Constant  Value=3650.2596024388
  Constant_3650.2596024388_c8e21 : Constant  Value=3650.2596024388
  Constant_376.991118430775_518d3 : Constant  Value=376.991118430775
  Product_33455 : Product
  Product_495fc : Product
  Product_5d224 : Product
  Product_bf27f : Product
  Subtract_ae73f : Sum  Inputs=+-
  Blockout_d_id_line_6_7_4abc2 : Outport
  wires:
  Constant_-45.1713972564836_0ad27/1 -> Product_bf27f/1
  Product_33455/1 -> Add_112c4/2
  State_id_line_6_7_fdc4e/1 -> Product_bf27f/2
  Constant_376.991118430775_518d3/1 -> Product_33455/1
  State_iq_line_6_7_9688a/1 -> Product_33455/2
  Product_bf27f/1 -> Add_112c4/1
  Constant_3650.2596024388_c2f5c/1 -> Product_495fc/1
  State_vd_bus_6_febc2/1 -> Product_495fc/2
  Add_112c4/1 -> Add_f2513/1
  Product_495fc/1 -> Add_f2513/2
  Constant_3650.2596024388_c8e21/1 -> Product_5d224/1
  State_vd_bus_7_50435/1 -> Product_5d224/2
  Add_f2513/1 -> Subtract_ae73f/1
  Product_5d224/1 -> Subtract_ae73f/2
  Subtract_ae73f/1 -> Blockout_d_id_line_6_7_4abc2/1

== system case1/AC_1/d_id_line_7_8_block ==
  note: d_id_line_7_8 in case1
      | $376.991118430775\,\mathrm{iq}_{\mathrm{line},7,8}-45.1713972564836\,\mathrm{id}_{\mathrm{line},7,8}+5110.36344341432\,\mathrm{vd}_{\mathrm{bus},7}-5110.36344341432\,\mathrm{vd}_{\mathrm{bus},8}$
      | Automatically generated on 2025-10-31 18:50:54 .
  State_id_line_7_8_8dd6f : Inport
  State_iq_line_7_8_d3a92 : Inport  Port=2
  State_vd_bus_7_5e09f : Inport  Port=3
  State_vd_bus_8_2c1e2 : Inport  Port=4
  Add_28665 : Sum
  Add_902df : Sum
  Constant_-45.1713972564836_682c8 : Constant  Value=-45.1713972564836
  Constant_376.991118430775_a6df8 : Constant  Value=376.991118430775
  Constant_5110.36344341432_da673 : Constant  Value=5110.36344341432
  Constant_5110.36344341432_fb380 : Constant  Value=5110.36344341432
  Product_4730c : Product
  Product_89f2f : Product
  Product_ec67d : Product
  Product_fe08a : Product
  Subtract_c126a : Sum  Inputs=+-
  Blockout_d_id_line_7_8_4d2a9 : Outport
  wires:
  Constant_-45.1713972564836_682c8/1 -> Product_89f2f/1
  Product_4730c/1 -> Add_902df/2
  State_id_line_7_8_8dd6f/1 -> Product_89f2f/2
  Constant_376.991118430775_a6df8/1 -> Product_4730c/1
  Product_89f2f/1 -> Add_902df/1
  State_iq_line_7_8_d3a92/1 -> Product_4730c/2
  Constant_5110.36344341432_fb380/1 -> Product_fe08a/1
  State_vd_bus_7_5e09f/1 -> Product_fe08a/2
  Add_902df/1 -> Add_28665/1
  Product_fe08a/1 -> Add_28665/2
  Constant_5110.36344341432_da673/1 -> Product_ec67d/1
  State_vd_bus_8_2c1e2/1 -> Product_ec67d/2
  Add_28665/1 -> Subtract_c126a/1
  Product_ec67d/1 -> Subtract_c126a/2
  Subtract_c126a/1 -> Blockout_d_id_line_7_8_4d2a9/1

== system case1/AC_1/d_id_line_8_2_block ==
  note: d_id_line_8_2 in case1
      | $376.991118430775\,\mathrm{iq}_{\mathrm{line},8,2}-5887.13868681329\,\mathrm{vd}_{\mathrm{bus},2}+5887.13868681329\,\mathrm{vd}_{\mathrm{bus},8}$
      | Automatically generated on 2025-10-31 18:50:56 .
  State_iq_line_8_2_ef0f1 : Inport
  State_vd_bus_2_8c8c2 : Inport  Port=2
  State_vd_bus_8_5928a : Inport  Port=3
  Add_3f326 : Sum
  Constant_376.991118430775_19e64 : Constant  Value=376.991118430775
  Constant_5887.13868681329_62aec : Constant  Value=5887.13868681329
  Constant_5887.13868681329_8cb2f : Constant  Value=5887.13868681329
  Product_303a8 : Product
  Product_b2e8d : Product
  Product_edbf5 : Product
  Subtract_c7914 : Sum  Inputs=+-
  Blockout_d_id_line_8_2_bde2e : Outport
  wires:
  State_vd_bus_2_8c8c2/1 -> Product_edbf5/2
  Constant_376.991118430775_19e64/1 -> Product_b2e8d/1
  Product_edbf5/1 -> Subtract_c7914/2
  State_iq_line_8_2_ef0f1/1 -> Product_b2e8d/2
  Constant_5887.13868681329_8cb2f/1 -> Product_edbf5/1
  Product_b2e8d/1 -> Subtract_c7914/1
  Constant_5887.13868681329_62aec/1 -> Product_303a8/1
  State_vd_bus_8_5928a/1 -> Product_303a8/2
  Subtract_c7914/1 -> Add_3f326/1
  Product_303a8/1 -> Add_3f326/2
  Add_3f326/1 -> Blockout_d_id_line_8_2_bde2e/1

== system case1/AC_1/d_id_line_8_9_block ==
  note: d_id_line_8_9 in case1
      | $376.991118430775\,\mathrm{iq}_{\mathrm{line},8,9}-76.0503465684605\,\mathrm{id}_{\mathrm{line},8,9}+2285.37992500516\,\mathrm{vd}_{\mathrm{bus},8}-2285.37992500516\,\mathrm{vd}_{\mathrm{bus},9}$
      | Automatically generated on 2025-10-31 18:50:58 .
  State_id_line_8_9_76f67 : Inport
  State_iq_line_8_9_c72f1 : Inport  Port=2
  State_vd_bus_8_54a05 : Inport  Port=3
  State_vd_bus_9_ba6dc : Inport  Port=4
  Add_49ee1 : Sum
  Add_efbba : Sum
  Constant_-76.0503465684605_c4e06 : Constant  Value=-76.0503465684605
  Constant_2285.37992500516_21757 : Constant  Value=2285.37992500516
  Constant_2285.37992500516_e467f : Constant  Value=2285.37992500516
  Constant_376.991118430775_8d362 : Constant  Value=376.991118430775
  Product_4499f : Product
  Product_6914b : Product
  Product_d54b8 : Product
  Product_ea52c : Product
  Subtract_879b6 : Sum  Inputs=+-
  Blockout_d_id_line_8_9_bdb89 : Outport
  wires:
  Constant_-76.0503465684605_c4e06/1 -> Product_6914b/1
  Product_d54b8/1 -> Add_49ee1/2
  State_id_line_8_9_76f67/1 -> Product_6914b/2
  Constant_376.991118430775_8d362/1 -> Product_d54b8/1
  State_iq_line_8_9_c72f1/1 -> Product_d54b8/2
  Product_6914b/1 -> Add_49ee1/1
  Constant_2285.37992500516_21757/1 -> Product_ea52c/1
  State_vd_bus_8_54a05/1 -> Product_ea52c/2
  Add_49ee1/1 -> Add_efbba/1
  Product_ea52c/1 -> Add_efbba/2
  Constant_2285.37992500516_e467f/1 -> Product_4499f/1
  State_vd_bus_9_ba6dc/1 -> Product_4499f/2
  Add_efbba/1 -> Subtract_879b6/1
  Product_4499f/1 -> Subtract_879b6/2
  Subtract_879b6/1 -> Blockout_d_id_line_8_9_bdb89/1

== system case1/AC_1/d_id_line_9_4_block ==
  note: d_id_line_9_4 in case1
      | $376.991118430775\,\mathrm{iq}_{\mathrm{line},9,4}-45.0150948438314\,\mathrm{id}_{\mathrm{line},9,4}-4328.77844618625\,\mathrm{vd}_{\mathrm{bus},4}+4328.77844618625\,\mathrm{vd}_{\mathrm{bus},9}$
      | Automatically generated on 2025-10-31 18:51:01 .
  State_id_line_9_4_23399 : Inport
  State_iq_line_9_4_9f86a : Inport  Port=2
  State_vd_bus_4_9315c : Inport  Port=3
  State_vd_bus_9_43177 : Inport  Port=4
  Add_2ff1d : Sum
  Add_d494a : Sum
  Constant_-45.0150948438314_8014b : Constant  Value=-45.0150948438314
  Constant_376.991118430775_c9160 : Constant  Value=376.991118430775
  Constant_4328.77844618625_2b251 : Constant  Value=4328.77844618625
  Constant_4328.77844618625_64db6 : Constant  Value=4328.77844618625
  Product_104e6 : Product
  Product_1a257 : Product
  Product_6318f : Product
  Product_86984 : Product
  Subtract_3598e : Sum  Inputs=+-
  Blockout_d_id_line_9_4_20edc : Outport
  wires:
  Constant_-45.0150948438314_8014b/1 -> Product_86984/1
  Product_6318f/1 -> Add_d494a/2
  State_id_line_9_4_23399/1 -> Product_86984/2
  Constant_376.991118430775_c9160/1 -> Product_6318f/1
  Product_86984/1 -> Add_d494a/1
  State_iq_line_9_4_9f86a/1 -> Product_6318f/2
  Constant_4328.77844618625_64db6/1 -> Product_104e6/1
  State_vd_bus_4_9315c/1 -> Product_104e6/2
  Add_d494a/1 -> Subtract_3598e/1
  Product_104e6/1 -> Subtract_3598e/2
  Constant_4328.77844618625_2b251/1 -> Product_1a257/1
  Subtract_3598e/1 -> Add_2ff1d/1
  State_vd_bus_9_43177/1 -> Product_1a257/2
  Product_1a257/1 -> Add_2ff1d/2
  Add_2ff1d/1 -> Blockout_d_id_line_9_4_20edc/1

== system case1/AC_1/d_id_load_5_block ==
  note: d_id_load_5 in case1
      | $376.991118430775\,\mathrm{iq}_{\mathrm{load},5}-1076.79807376298\,\mathrm{id}_{\mathrm{load},5}+1165.56205079599\,\mathrm{vd}_{\mathrm{bus},5}$
      | Automatically generated on 2025-10-31 18:50:36 .
  State_id_load_5_a7934 : Inport
  State_iq_load_5_1055a : Inport  Port=2
  State_vd_bus_5_1aa4f : Inport  Port=3
  Add_5fbf6 : Sum
  Add_a749a : Sum
  Constant_-1076.79807376298_d4bcf : Constant  Value=-1076.79807376298
  Constant_1165.56205079599_250dd : Constant  Value=1165.56205079599
  Constant_376.991118430775_25eb9 : Constant  Value=376.991118430775
  Product_0002e : Product
  Product_310b3 : Product
  Product_f7031 : Product
  Blockout_d_id_load_5_7c560 : Outport
  wires:
  Constant_-1076.79807376298_d4bcf/1 -> Product_f7031/1
  Product_310b3/1 -> Add_5fbf6/2
  State_id_load_5_a7934/1 -> Product_f7031/2
  Constant_376.991118430775_25eb9/1 -> Product_310b3/1
  Product_0002e/1 -> Add_a749a/2
  State_iq_load_5_1055a/1 -> Product_310b3/2
  Product_f7031/1 -> Add_5fbf6/1
  Constant_1165.56205079599_250dd/1 -> Product_0002e/1
  State_vd_bus_5_1aa4f/1 -> Product_0002e/2
  Add_5fbf6/1 -> Add_a749a/1
  Add_a749a/1 -> Blockout_d_id_load_5_7c560/1
